simulink model "Inverter_H_Bridge"  (R2018a)
settings: Solver=VariableStepAuto  StartTime=0.0  StopTime=1  RelTol=1e-3
libraries: powerlib x10
settings Model: Creator=ozie  LastModifiedBy=ozie

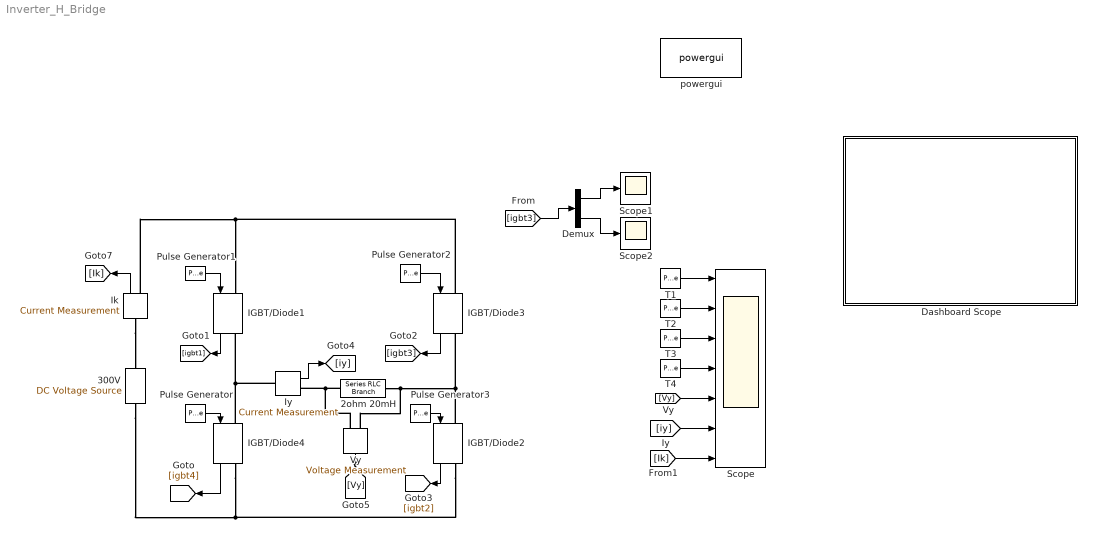
== system Inverter_H_Bridge ==
  2ohm 20mH : powerlib/Elements/Series RLC Branch  LConnTagsString=__new0  RConnTagsString=__new0  BranchType=RL  Resistance=2  Inductance=20e-3  SetiL0=off  InitialCurrent=0  Capacitance=1e-6  Setx0=off  InitialVoltage=0  Measurements=None
  300V : powerlib/Electrical Sources/DC Voltage Source  Amplitude=300  Measurements=None
  Dashboard Scope : Subsystem  DialogController=hmiCreateDDGDialog  IsWebBlock=on  mask(MWDashboardBlock){webBlockId=ea89e24b-939d-4496-9d35-2949cdf7117a, webBlockType=sdiscope, ShowInitialText=on, HMISrcModelName=Inverter_H_Bridge}
      mask prompts: webBlockId "WebBlock Id"; webBlockType "WebBlock Type"; HMISrcModelName "Source Model"
      mask help: SimulinkHMI:dialogs:HMIScopeDialogDesc
      mask Help: helpview([docroot '/mapfiles/simulink.map'], 'hmi_scope')
      mask Display:
      | if strcmp(get_param(bdroot(gcb),'BlockDiagramType'), 'library')
      |     image([(matlabroot) '/toolbox/simulink/hmi/icons/DashboardScope.png']);
      | end
  Demux : Demux  Outputs=2
  IGBT/Diode{1..4} (4 alike) : powerlib/Power Electronics/IGBT//Diode  Ron=1e-3  Rs=1e5  Cs=inf  Measurements=on
  Ik : powerlib/Measurements/Current Measurement  PhasorSimulation=off  OutputType=Complex  PSBequivalent=0
  Iy : powerlib/Measurements/Current Measurement  PhasorSimulation=off  OutputType=Complex  PSBequivalent=0
  Pulse Generator : DiscretePulseGenerator  PulseType=Time based  Period=1/60  PulseWidth=50  PhaseDelay=0.0083*(96.8/180)
  Pulse Generator1 : DiscretePulseGenerator  PulseType=Time based  Period=1/60  PulseWidth=50  PhaseDelay=0.0083*(-83.2/180)
  Pulse Generator2 : DiscretePulseGenerator  PulseType=Time based  Period=1/60  PulseWidth=50  PhaseDelay=0.0083*(180/180)
  Pulse Generator3 : DiscretePulseGenerator  PulseType=Time based  Period=1/60  PulseWidth=50  PhaseDelay=0.0083*(0/180)
  Scope : Scope  NumInputPorts=7
  Scope1 : Scope
  Scope2 : Scope
  T1 : DiscretePulseGenerator  PulseType=Time based  Period=1/60  PulseWidth=50  PhaseDelay=0.0083*(-83.2/180)
  T2 : DiscretePulseGenerator  PulseType=Time based  Period=1/60  PulseWidth=50  PhaseDelay=0.0083*(0/180)
  T3 : DiscretePulseGenerator  PulseType=Time based  Period=1/60  PulseWidth=50  PhaseDelay=0.0083*(180/180)
  T4 : DiscretePulseGenerator  PulseType=Time based  Period=1/60  PulseWidth=50  PhaseDelay=0.005*(96.8/180)
  "Vy " : powerlib/Measurements/Voltage Measurement  PhasorSimulation=off  OutputType=Complex  PSBequivalent=0
  powergui : powerlib/powergui  Priority=1  SimulationMode=Continuous  SampleTime=50e-6  frequency=60  Iterations=50  frequencyindice=0  Pbase=100e6  ErrMax=1e-4  UnitsV=kV  UnitsW=MW  buscounter=0  FunctionMessages=off  echomessages=off  EnableUseOfTLC=off  CurrentSourceSwitches=off  DisableSnubberDevices=off  DisableRonSwitches=off  DisableVfSwitches=off  DisplayEquations=off  SolverType=Tustin/Backward Euler (TBE)  Interpol=off  ExternalGateDelay=off  methode=off  Ts=100  x0status=blocks  SPID=on  SwTol=0  HookPort=off  RestoreLinks=warning  ResistiveCurrentMeasurement=off  Frange=[0:2:500]  Ylog=off  Xlog=on  ShowGrid=off  save=off  variable=ZData  structure=logsout  ZoomFFT=off  StartTime=0.0  cycles=1  DisplayStyle=1  fundamental=60  FreqAxis=off  MaxFrequency=1000  frequencyindicesteady=1  RmsSteady=1  display=off
  wires:
  Pulse Generator/1 -> IGBT/Diode4/1
  Pulse Generator1/1 -> IGBT/Diode1/1
  Pulse Generator2/1 -> IGBT/Diode3/1
  Pulse Generator3/1 -> IGBT/Diode2/1
  Iy/1 -> [iy]
  "Vy "/1 -> [Vy]
  T1/1 -> Scope/1
  T3/1 -> Scope/3
  T4/1 -> Scope/4
  [Vy] -> Scope/5
  [iy] -> Scope/6
  Ik/1 -> [Ik]
  T2/1 -> Scope/2
  IGBT/Diode4/1 -> [igbt4]
  IGBT/Diode1/1 -> [igbt1]
  IGBT/Diode3/1 -> [igbt3]
  IGBT/Diode2/1 -> [igbt2]
  [Ik] -> Scope/7
  Demux/1 -> Scope1/1
  Demux/2 -> Scope2/1
  [igbt3] -> Demux/1
  connections:
  2ohm 20mH/LConn1 -- "Vy "/LConn1 -- Iy/RConn1
  2ohm 20mH/RConn1 -- "Vy "/LConn2 -- IGBT/Diode2/LConn1 -- IGBT/Diode3/RConn1
  Ik/LConn1 -- 300V/RConn1
  300V/LConn1 -- IGBT/Diode2/RConn1 -- IGBT/Diode4/RConn1
  Iy/LConn1 -- IGBT/Diode4/LConn1 -- IGBT/Diode1/RConn1
  Ik/RConn1 -- IGBT/Diode3/LConn1 -- IGBT/Diode1/LConn1

== system Inverter_H_Bridge/Dashboard Scope ==
